simulink model "model"  (R2020b)
settings: Solver=FixedStepAuto  StartTime=0.0  StopTime=inf  FixedStep=0.5  RelTol=1e-3  EnableMultiTasking=on
libraries: arduinolib x2, simulink x2, pid_lib x1
settings Model: SILPILModeSetting=veronly  ExtModeTrigDuration=2  Creator=Reginald Nyakonda  LastModifiedBy=Reginald Nyakonda
settings OptimizationCC: EnhancedBackFolding=on  PassReuseOutputArgsAs=Individual arguments  ZeroExternalMemoryAtStartup=off  ZeroInternalMemoryAtStartup=off  MaxStackSize=64  OptimizeBlockOrder=speed  DifferentSizesBufferReuse=on  EfficientTunableParamExpr=on
settings DebuggingCC: ParameterTunabilityLossMsg=error
settings HardwareCC: ProdBitPerInt=16  ProdBitPerPointer=16  ProdBitPerSizeT=16  ProdBitPerPtrDiffT=16  ProdLargestAtomicFloat=None  ProdWordSize=8  ProdHWDeviceType=Atmel->AVR  UseEmbeddedCoderFeatures=off  UseSimulinkCoderFeatures=off
settings SFSimCC: MATLABDynamicMemAlloc=off
settings RTWCC: Description=Embedded Coder  SystemTargetFile=ert.tlc  HardwareBoard=Arduino Mega 2560  TemplateMakefile=ert_default_tmf  Toolchain=Arduino AVR  BuildConfiguration=Faster Runs
settings CodeAppCC: ForceParamTrailComments=on  IgnoreCustomStorageClasses=off  OperatorAnnotations=on  SimulinkDataObjDesc=on  SFDataObjDesc=on  InsertBlockDesc=on
settings ERTTargetCC: SupportContinuousTime=on  SupportNonInlinedSFcns=on  SupportVariableSizeSignals=on  ExtModeStaticAllocSize=2048

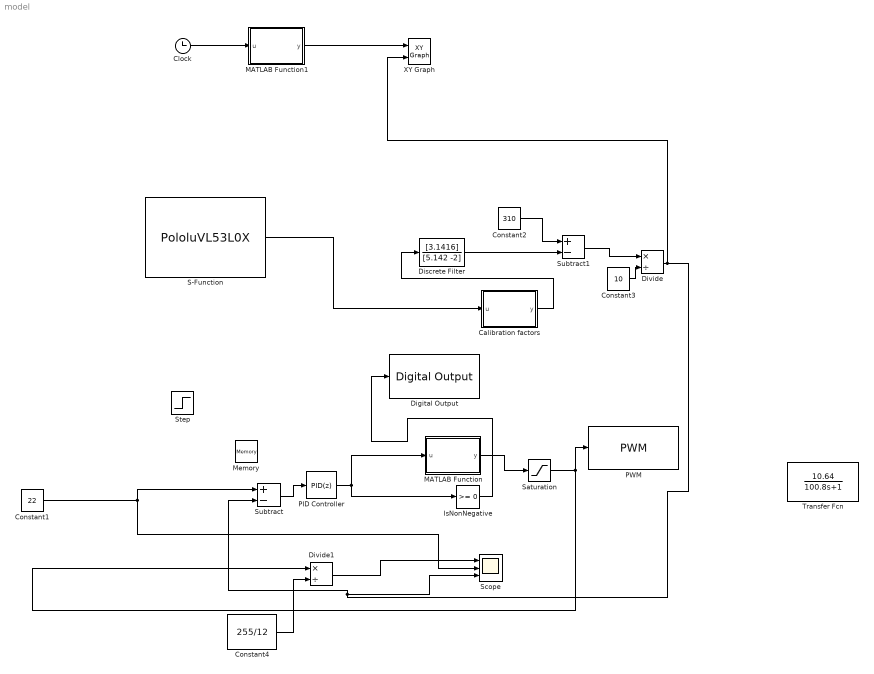
== system model ==
  Calibration factors : MATLAB Function  TreatAsAtomicUnit=on
  Clock : Clock
  Constant1 : Constant  Value=22
  Constant2 : Constant  Value=310
  Constant3 : Constant  Value=10
  Constant4 : Constant  Value=255/12
  Digital Output : arduinolib/Digital Output  pinNumber=12  Direction=output  blockPlatform=arduino
  Discrete Filter : DiscreteFilter  Numerator=[3.1416]  Denominator=[5.142 -2]
  Divide : Product  Inputs=*/
  Divide1 : Product  Inputs=*/
  IsNonNegative : simulink/Logic and Bit Operations/Compare To Zero  relop=>=  OutDataTypeStr=boolean
  MATLAB Function : MATLAB Function  TreatAsAtomicUnit=on
  MATLAB Function1 : MATLAB Function  TreatAsAtomicUnit=on
  Memory : Memory
  PID Controller : pid_lib/PID Controller  Controller=PID  Form=Parallel  TimeDomain=Discrete-time  UseExternalTs=off  SampleTime=-1  IntegratorMethod=Forward Euler  FilterMethod=Forward Euler  ControllerParametersSource=internal  P=0.9138  I=0.0223  D=-1.917  UseFilter=on  N=0.0614  TunerSelectOption=Transfer Function Based (PID Tuner App)  InitialConditionSource=internal  InitialConditionForIntegrator=0  InitialConditionForFilter=0  DifferentiatorICPrevScaledInput=0  ExternalReset=none  TrackingMode=off  Kt=1  LimitOutput=on  SatLimitsSource=internal  UpperSaturationLimit=255  LowerSaturationLimit=0  LinearizeAsGain=on  AntiWindupMode=clamping  Kb=1  POutMin=[]  POutMax=[]  IOutMin=[]  IOutMax=[]  DOutMin=[]  DOutMax=[]  NOutMin=[]  NOutMax=[]  SumOutMin=[]  SumOutMax=[]  SaturationOutMin=[]  SaturationOutMax=[]  PParamMin=[]  PParamMax=[]  IParamMin=[]  IParamMax=[]  DParamMin=[]  DParamMax=[]  NParamMin=[]  NParamMax=[]  KbParamMin=[]  KbParamMax=[]  KtParamMin=[]  KtParamMax=[]  KbOutMin=[]  KbOutMax=[]  KtOutMin=[]  KtOutMax=[]  IntegratorOutMin=[]  IntegratorOutMax=[]  FilterOutMin=[]  FilterOutMax=[]  SumI1OutMin=[]  SumI1OutMax=[]  SumI2OutMin=[]  SumI2OutMax=[]  SumI3OutMin=[]  SumI3OutMax=[]  SumI4OutMin=[]  SumI4OutMax=[]  SumDOutMin=[]  SumDOutMax=[]  DifferentiatorOutMin=[]  DifferentiatorOutMax=[]  FilterDiffOutCoefMin=[]  FilterDiffOutCoefMax=[]  ReciprocalOutMin=[]  ReciprocalOutMax=[]  SumDenOutMin=[]  SumDenOutMax=[]  SumNumOutMin=[]  SumNumOutMax=[]  DivideOutMin=[]  DivideOutMax=[]  UdiffTsProdOutMin=[]  UdiffTsProdOutMax=[]  NTsProdOutMin=[]  NTsProdOutMax=[]  UintegralTsProdOutMin=[]  UintegralTsProdOutMax=[]  UngainTsProdOutMin=[]  UngainTsProdOutMax=[]  IntegratorContinuousStateAttributes=''  IntegratorStateMustResolveToSignalObject=off  IntegratorRTWStateStorageClass=Auto  FilterContinuousStateAttributes=''  FilterStateMustResolveToSignalObject=off  FilterRTWStateStorageClass=Auto  ParallelPVariant=InternalParameters  IdealPVariant=Disabled  IVariant=InternalParameters  DVariant=InternalParameters  IntegratorVariant=Discrete  SatVariant=Enabled  AWVariant=DiscClampingParallel  PCopyVariant=Disabled  TRVariant=Disabled  FdbkBlocksVariant=Forward  IdealPFdbkVariant=Disabled  SatFdbkVariant=Disabled  DerivativeFilterVariant=ForwardEulerFilter  NVariant=InternalParameters  NCopyVariant=Disabled  FilterICVariant=InternalICsFilter  IntegratorICVariant=InternalICs  ExternalResetVariant=Disabled  TRSumVariant=Passthrough  SumFdbkVariant=Disabled  SumVariant=Sum_PID  TsampFilterVariant=InternalTs  TsampNgainVariant=Passthrough  TsampIntegralVariant=Passthrough  ExternalSaturationOutDataTypeStr=Inherit: Same as second input
  PWM : arduinolib/PWM  pinNumber=10  frequencyType=Default  desiredFrequency=490.2  achievableFrequency=490.2
  S-Function : S-Function  FunctionName=PololuVL53L0X  SFunctionModules=PololuVL53L0X_wrapper  SFunctionDeploymentMode=off  EnableBusSupport=off
  Saturation : Saturate  UpperLimit=255  LowerLimit=0
  Scope : Scope  NumInputPorts=3
  Step : Step  Time=10  After=120  SampleTime=0.5
  Subtract : Sum  Inputs=+-
  Subtract1 : Sum  Inputs=+-
  Transfer Fcn : TransferFcn  Numerator=[10.64]  Denominator=[100.8 1]
  XY Graph : simulink/Sinks/XY Graph  xmin=0  xmax=1500  ymin=0  ymax=35  st=-1
  wires:
  S-Function/1 -> Calibration factors/1(u)
  IsNonNegative/1 -> Digital Output/1
  Constant2/1 -> Subtract1/1
  Subtract1/1 -> Divide/1
  Constant3/1 -> Divide/2
  PID Controller/1 -> MATLAB Function/1(u), IsNonNegative/1
  Calibration factors/1(y) -> Discrete Filter/1
  MATLAB Function/1(y) -> Saturation/1
  Saturation/1 -> PWM/1, Divide1/1
  Divide/1 -> XY Graph/2, Subtract/2, Scope/3
  Constant4/1 -> Divide1/2
  Divide1/1 -> Scope/1
  Constant1/1 -> Subtract/1, Scope/2
  Discrete Filter/1 -> Subtract1/2
  Subtract/1 -> PID Controller/1
  Clock/1 -> MATLAB Function1/1(u)
  MATLAB Function1/1(y) -> XY Graph/1

== matlab function model/Calibration factors ==
  data: u input; y output
function y = fcn(u)
if u>=10 && u<=60
    output = u*1.06;
elseif u>60 && u<=130
    output = u*1.12;
elseif u>130 && u<=150
    output = u;
elseif u>150 && u<=270
    output = u*0.92;
    
elseif u>270 && u<=330
    output = u*0.98;
else
    output = 305;
end    
y = output;

== matlab function model/MATLAB Function1 ==
  data: u input; y output
function y = fcn(u)
volume = u*10.5;
y = volume;

== matlab function model/MATLAB Function ==
  data: u input; y output
function y = fcn(u)
if u<0
    u = 0;
else
    u=abs(u);
end

y = u;
